simulink model "B_dot"  (Simulink 7.4)
settings: Solver=ode45  StartTime=0.0  StopTime=150000.0  RelTol=1e-3
libraries: aausat3_lib x8
settings Model: Creator=KFJensen  LastModifiedBy=kasperv
settings DataIOCC: LimitDataPoints=off
settings OptimizationCC: InlineParams=on  SimCompilerOptimization=On
settings DebuggingCC: SignalInfNanChecking=error  IntegerOverflowMsg=error  ParameterUnderflowMsg=error  AssertControl=DisableAll  StrictBusMsg=None
settings HardwareCC: ProdHWDeviceType=Generic->Unspecified (assume 32-bit Generic)

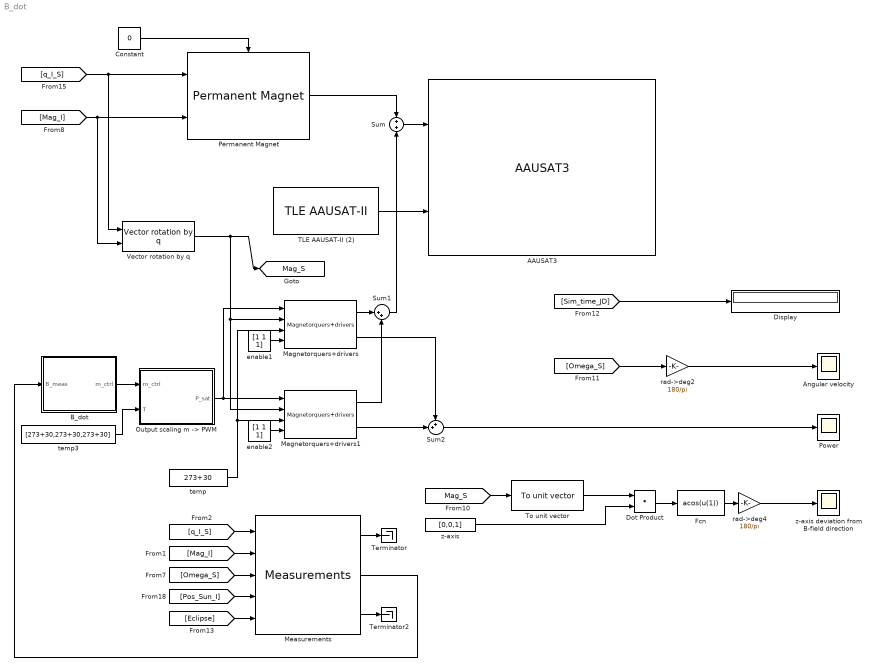
== system B_dot ==
  AAUSAT3 : aausat3_lib/AAUSAT3  SystemSampleTime=-1  r_com_s=[0.049073,0.048909,0.042976]  sat_temp_start=293.15  mass_sc=0.957820  Dim=[0.1,0.1,0.11]  inertia_c=[0.0017464,0.0022092,0.0022388]  init_jd=2455153.1954318  q_s_c=[-0.020656,0.71468,-0.007319,0.6991]  q_init_I_S=[1 0 0 0]  w_init_s=[1,1,1]*10*pi/180  Cd=2  rho=5e-14  solar_m_flux=4.5565e-6  solar_absorb_coeff=1.5  theta_e=65  refldata=load('lib/AlbedoToolbox-1.0/refl_data/2005/ga050101-051231')  redfac=1  Ts=1  enable_sensor_emulation=on  enable_env_disturbance=on
  Angular velocity : Scope
      settings: TimeRange=48000  YMin=-1  YMax=1  SaveName=ScopeData2  SampleInput=on
  B_dot : Subsystem  AncestorBlock=aausat3_lib/ACS/B_dot  mask{C=6000, wc=0.7, m_pm=-0.0030, Ts=0.1}
      mask prompts: C "Gain:"; wc "Filter cutoff frequency:"; m_pm "Permanent magnet dipole moment:"; Ts "Sample time:"
  Constant : Constant  Value=0  OutDataType=fixdt(1, 16)  OutScaling=2^0
  Display : Display
  Dot Product : DotProduct  OutDataType=fixdt(1, 16)  OutScaling=2^-10  InputSameDT=on  OutDataTypeStr=Inherit: Inherit via internal rule
  Fcn : Fcn  Expr=acos(u(1))
  Magnetorquers+drivers : aausat3_lib/Actuator Emulation/Magnetorquers+drivers  SystemSampleTime=-1  coil_dim=[0.075,0.075]  n_mt=250  A_wire_mt=(pi/4)*(0.13e-3)^2  sigma_0_mt=1.7e-8  alpha_0_mt=3.9e-3  T_0_mt=293.15  freq_mag=10  duty_mag=88
  Magnetorquers+drivers1 : aausat3_lib/Actuator Emulation/Magnetorquers+drivers  SystemSampleTime=-1  coil_dim=[0.075,0.075]  n_mt=250  A_wire_mt=(pi/4)*(0.13e-3)^2  sigma_0_mt=1.7e-8  alpha_0_mt=3.9e-3  T_0_mt=293.15  freq_mag=10  duty_mag=88
  Measurements : aausat3_lib/Sensor Emulation/Measurements  SystemSampleTime=-1  s_freq_mag=10  noise_mag=3  bias_mag=[0 0 0]  heading_mag=0  tilt_mag=0  s_freq_sun=1  noise_sun=3.33  bias_sun=[0 0]  nr_sample_sun=1  s_freq_gyro=1  noise_gyro=0.2  bias_gyro=[0 0 0]  heading_gyro=0  tilt_gyro=0
  "Output scaling m -> PWM" : Subsystem  AncestorBlock=aausat3_lib/Actuator Emulation/Output scaling m -> PWM  mask{coil_dim=[0.075,0.075], n_mt=250, A_wire_mt=(pi/4)*(0.13e-3)^2, sigma_0_mt=1.7e-8, alpha_0_mt=3.9e-3, T_0_mt=293.15, PWM_max=62.5, PWM_min=37.5}
      mask prompts: coil_dim "Coil Dimensions [x,y][m]:"; n_mt "Coil Winding Number [-]:"; A_wire_mt "Wire Cross Sectional Area [m^2]:"; sigma_0_mt "Wire Resistivity [Ohm*m]:"; alpha_0_mt "Wire Resistivity Temperature Coefficient [(deg C)^-1]:"; T_0_mt "Wire Resistivity Base Temperature [K]:"; PWM_max "PWM max [%]"; PWM_min "PWM min [%]"
  Permanent Magnet : aausat3_lib/Actuator Emulation/Permanent Magnet  SystemSampleTime=-1  mag_moment=-0.0030
  Power : Scope
      settings: TimeRange=48000  YMin=0  YMax=0.035  SaveName=ScopeData3  SampleInput=on
  Sum : Sum  OutDataType=fixdt(1, 16)  OutScaling=2^0
  Sum1 : Sum  Inputs=|++  OutDataType=fixdt(1, 16)  OutScaling=2^0
  Sum2 : Sum  Inputs=++|  OutDataType=fixdt(1, 16)  OutScaling=2^0
  TLE AAUSAT-II (2) : aausat3_lib/Orbit and Ephemeris/TLE AAUSAT-II  SystemSampleTime=-1  satname='AAUSAT-II'  JulianDay=09321.69542252  xndt2o=0.00000555  xndd6o=0.0  bstar=.76898e-4  xincl=97.9251  xnodeo=24.1597  eo=0.0014245  omegao=254.1774  xmo=105.7862  xno=14.81823818  ts=1
  Terminator : Terminator
  Terminator2 : Terminator
  To unit vector : aausat3_lib/Math Utilities/Vector operations/To unit vector  SystemSampleTime=-1
  Vector rotation by q : aausat3_lib/Actuator Emulation/Permanent Magnet/Vector rotation by q  SystemSampleTime=-1
  enable1 : Constant  Value=[1 1 1]  OutDataType=fixdt(1, 16)  OutScaling=2^0
  enable2 : Constant  Value=[1 1 1]  VectorParams1D=off  OutDataType=fixdt(1, 16)  OutScaling=2^0
  rad->deg2 : Gain  Gain=180/pi  ParameterDataType=fixdt(1, 16)  ParameterScaling=2^0  OutDataType=fixdt(1, 16)  OutScaling=2^0
  rad->deg4 : Gain  Gain=180/pi  ParameterDataType=fixdt(1, 16)  ParameterScaling=2^0  OutDataType=fixdt(1, 16)  OutScaling=2^0
  temp : Constant  Value=273+30  OutDataType=fixdt(1, 16)  OutScaling=2^0
  temp3 : Constant  Value=[273+30,273+30,273+30]  OutDataType=fixdt(1, 16)  OutScaling=2^0
  z-axis : Constant  Value=[0,0,1]  OutDataType=fixdt(1, 16)  OutScaling=2^0
  z-axis deviation from B-field direction : Scope
      settings: TimeRange=48000  YMin=0  YMax=180  SaveName=ScopeData9  SampleInput=on  SampleTime=1
  tag scope: Mag_S=global
  wires:
  TLE AAUSAT-II (2)/1 -> AAUSAT3/2
  [q_I_S] -> Permanent Magnet/1, Vector rotation by q/1
  [Mag_I] -> Permanent Magnet/2, Vector rotation by q/2
  Constant/1 -> Permanent Magnet/Enable
  [q_I_S] -> Measurements/1
  [Mag_I] -> Measurements/2
  [Omega_S] -> Measurements/3
  [Sim_time_JD] -> Display/1
  [Eclipse] -> Measurements/5
  [Pos_Sun_I] -> Measurements/4
  Sum/1 -> AAUSAT3/1
  Measurements/1 -> Terminator/1
  Measurements/3 -> Terminator2/1
  Permanent Magnet/1 -> Sum/1
  [Omega_S] -> rad->deg2/1
  rad->deg2/1 -> Angular velocity/1
  Sum1/1 -> Sum/2
  Vector rotation by q/1 -> [Mag_S], Magnetorquers+drivers/2, Magnetorquers+drivers1/2
  B_dot/1(m_ctrl) -> "Output scaling m -> PWM"/1(m_ctrl)
  "Output scaling m -> PWM"/1(P_sat) -> Magnetorquers+drivers/1, Magnetorquers+drivers1/1
  enable1/1 -> Magnetorquers+drivers/4
  enable2/1 -> Magnetorquers+drivers1/4
  temp/1 -> Magnetorquers+drivers/3, Magnetorquers+drivers1/3
  temp3/1 -> "Output scaling m -> PWM"/2(T)
  Magnetorquers+drivers/1 -> Sum1/1
  Magnetorquers+drivers1/1 -> Sum1/2
  Measurements/2 -> B_dot/1(B_meas)
  Magnetorquers+drivers1/2 -> Sum2/2
  Magnetorquers+drivers/2 -> Sum2/1
  Sum2/1 -> Power/1
  z-axis/1 -> Dot Product/2
  Dot Product/1 -> Fcn/1
  Fcn/1 -> rad->deg4/1
  rad->deg4/1 -> z-axis deviation from B-field direction/1
  To unit vector/1 -> Dot Product/1
  [Mag_S] -> To unit vector/1

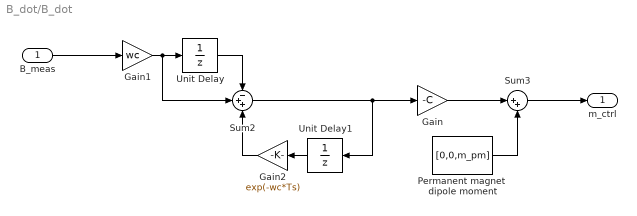
== system B_dot/B_dot ==
  B_meas : Inport  OutDataType=sfix(16)  OutScaling=2^0
  Gain : Gain  Gain=-C  ParameterDataType=fixdt(1, 16)  ParameterScaling=2^0  OutDataType=fixdt(1, 16)  OutScaling=2^0
  Gain1 : Gain  Gain=wc  ParameterDataType=fixdt(1, 16)  ParameterScaling=2^0  OutDataType=fixdt(1, 16)  OutScaling=2^0
  Gain2 : Gain  Gain=exp(-wc*Ts)  ParameterDataType=fixdt(1, 16)  ParameterScaling=2^0  OutDataType=fixdt(1, 16)  OutScaling=2^0
  Permanent magnet  dipole moment : Constant  Value=[0,0,m_pm]  OutDataType=fixdt(1, 16)  OutScaling=2^0
  Sum2 : Sum  Inputs=-++  OutDataType=fixdt(1, 16)  OutScaling=2^0
  Sum3 : Sum  Inputs=|++  OutDataType=fixdt(1, 16)  OutScaling=2^0
  Unit Delay : UnitDelay  SampleTime=-1
  Unit Delay1 : UnitDelay  SampleTime=-1
  m_ctrl : Outport  PortDimensions=3  OutDataType=sfix(16)  OutScaling=2^0
  wires:
  Sum3/1 -> m_ctrl/1
  Gain/1 -> Sum3/1
  Permanent magnet  dipole moment/1 -> Sum3/2
  Sum2/1 -> Unit Delay1/1, Gain/1
  Unit Delay1/1 -> Gain2/1
  Gain2/1 -> Sum2/3
  Gain1/1 -> Sum2/2, Unit Delay/1
  Unit Delay/1 -> Sum2/1
  B_meas/1 -> Gain1/1

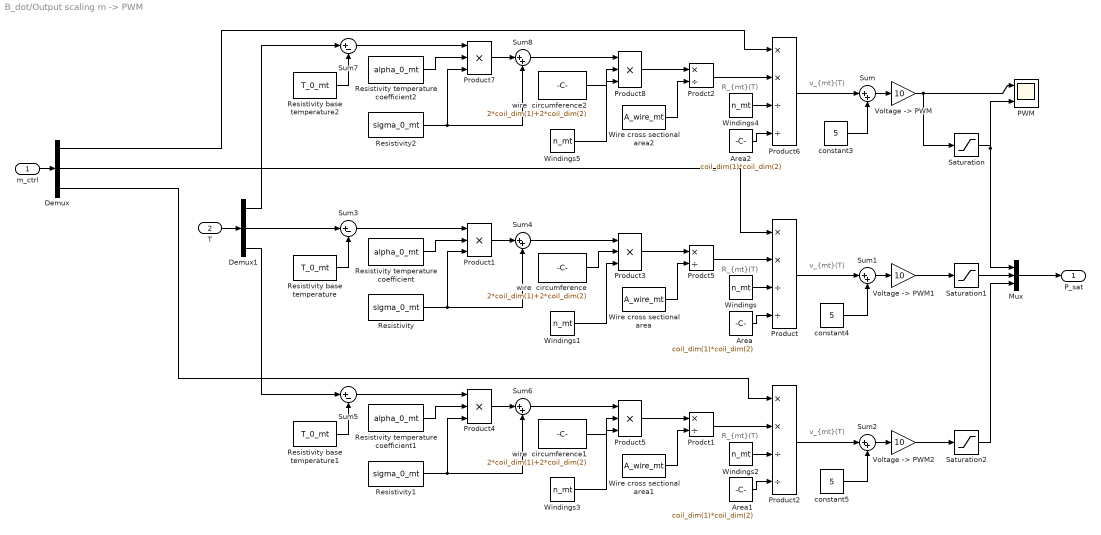
== system B_dot/Output scaling m -> PWM ==
  note: v_{mt}(T)
  note: v_{mt}(T)
  note: v_{mt}(T)
  note: R_{mt}(T)
  note: R_{mt}(T)
  note: R_{mt}(T)
  m_ctrl : Inport  OutDataType=sfix(16)  OutScaling=2^0
  T : Inport  Port=2  OutDataType=sfix(16)  OutScaling=2^0
  Area : Constant  Value=coil_dim(1)*coil_dim(2)  OutDataType=sfix(16)  OutScaling=2^0
  Area1 : Constant  Value=coil_dim(1)*coil_dim(2)  OutDataType=sfix(16)  OutScaling=2^0
  Area2 : Constant  Value=coil_dim(1)*coil_dim(2)  OutDataType=sfix(16)  OutScaling=2^0
  Demux : Demux  Outputs=3
  Demux1 : Demux  Outputs=3
  Mux : Mux  Inputs=3
  PWM : Scope  NumInputPorts=2
      settings: TimeRange=5000  YMin=37.5~37.5  YMax=67.5~62.5  SaveName=ScopeData4  SampleInput=on
  Prodct1 : Product  Inputs=*/  OutDataType=sfix(16)  OutScaling=2^0  RndMeth=Zero
  Prodct2 : Product  Inputs=*/  OutDataType=sfix(16)  OutScaling=2^0  RndMeth=Zero
  Prodct5 : Product  Inputs=*/  OutDataType=sfix(16)  OutScaling=2^0  RndMeth=Zero
  Product : Product  Inputs=**//  OutDataType=sfix(16)  OutScaling=2^0  RndMeth=Zero
  Product{1,3..5,7..8} (6 alike) : Product  Inputs=3  OutDataType=sfix(16)  OutScaling=2^0  RndMeth=Zero
  Product2 : Product  Inputs=**//  OutDataType=sfix(16)  OutScaling=2^0  RndMeth=Zero
  Product6 : Product  Inputs=**//  OutDataType=sfix(16)  OutScaling=2^0  RndMeth=Zero
  Resistivity : Constant  Value=sigma_0_mt  OutDataType=sfix(16)  OutScaling=2^0
  Resistivity base temperature : Constant  Value=T_0_mt  OutDataType=sfix(16)  OutScaling=2^0
  Resistivity base temperature1 : Constant  Value=T_0_mt  OutDataType=sfix(16)  OutScaling=2^0
  Resistivity base temperature2 : Constant  Value=T_0_mt  OutDataType=sfix(16)  OutScaling=2^0
  Resistivity temperature coefficient : Constant  Value=alpha_0_mt  OutDataType=sfix(16)  OutScaling=2^0
  Resistivity temperature coefficient1 : Constant  Value=alpha_0_mt  OutDataType=sfix(16)  OutScaling=2^0
  Resistivity temperature coefficient2 : Constant  Value=alpha_0_mt  OutDataType=sfix(16)  OutScaling=2^0
  Resistivity1 : Constant  Value=sigma_0_mt  OutDataType=sfix(16)  OutScaling=2^0
  Resistivity2 : Constant  Value=sigma_0_mt  OutDataType=sfix(16)  OutScaling=2^0
  Saturation : Saturate  UpperLimit=PWM_max  LowerLimit=PWM_min
  Saturation1 : Saturate  UpperLimit=PWM_max  LowerLimit=PWM_min
  Saturation2 : Saturate  UpperLimit=PWM_max  LowerLimit=PWM_min
  Sum : Sum  Inputs=|++  OutDataType=fixdt(1, 16)  OutScaling=2^0
  Sum1 : Sum  Inputs=|++  OutDataType=fixdt(1, 16)  OutScaling=2^0
  Sum2 : Sum  Inputs=|++  OutDataType=fixdt(1, 16)  OutScaling=2^0
  Sum3 : Sum  Inputs=|+-  OutDataType=sfix(16)  OutScaling=2^0
  Sum4 : Sum  Inputs=|++  OutDataType=sfix(16)  OutScaling=2^0
  Sum5 : Sum  Inputs=|+-  OutDataType=sfix(16)  OutScaling=2^0
  Sum6 : Sum  Inputs=|++  OutDataType=sfix(16)  OutScaling=2^0
  Sum7 : Sum  Inputs=|+-  OutDataType=sfix(16)  OutScaling=2^0
  Sum8 : Sum  Inputs=|++  OutDataType=sfix(16)  OutScaling=2^0
  "Voltage -> PWM" : Gain  Gain=10  ParameterDataType=fixdt(1, 16)  ParameterScaling=2^0  OutDataType=fixdt(1, 16)  OutScaling=2^0
  "Voltage -> PWM1" : Gain  Gain=10  ParameterDataType=fixdt(1, 16)  ParameterScaling=2^0  OutDataType=fixdt(1, 16)  OutScaling=2^0
  "Voltage -> PWM2" : Gain  Gain=10  ParameterDataType=fixdt(1, 16)  ParameterScaling=2^0  OutDataType=fixdt(1, 16)  OutScaling=2^0
  Windings{,1..5} (6 alike) : Constant  Value=n_mt  OutDataType=sfix(16)  OutScaling=2^0
  Wire cross sectional area : Constant  Value=A_wire_mt  OutDataType=sfix(16)  OutScaling=2^0
  Wire cross sectional area1 : Constant  Value=A_wire_mt  OutDataType=sfix(16)  OutScaling=2^0
  Wire cross sectional area2 : Constant  Value=A_wire_mt  OutDataType=sfix(16)  OutScaling=2^0
  constant3 : Constant  Value=5  OutDataType=sfix(16)  OutScaling=2^0
  constant4 : Constant  Value=5  OutDataType=sfix(16)  OutScaling=2^0
  constant5 : Constant  Value=5  OutDataType=sfix(16)  OutScaling=2^0
  wire  circumference : Constant  Value=2*coil_dim(1)+2*coil_dim(2)  OutDataType=sfix(16)  OutScaling=2^0
  wire  circumference1 : Constant  Value=2*coil_dim(1)+2*coil_dim(2)  OutDataType=sfix(16)  OutScaling=2^0
  wire  circumference2 : Constant  Value=2*coil_dim(1)+2*coil_dim(2)  OutDataType=sfix(16)  OutScaling=2^0
  P_sat : Outport  PortDimensions=3  OutDataType=sfix(16)  OutScaling=2^0
  wires:
  Product2/1 -> Sum2/1
  Product/1 -> Sum1/1
  Product6/1 -> Sum/1
  Demux/3 -> Product2/1
  Demux/2 -> Product/1
  Demux/1 -> Product6/1
  "Voltage -> PWM2"/1 -> Saturation2/1
  "Voltage -> PWM1"/1 -> Saturation1/1
  "Voltage -> PWM"/1 -> Saturation/1, PWM/1
  Area2/1 -> Product6/4
  Windings4/1 -> Product6/3
  Area1/1 -> Product2/4
  Windings2/1 -> Product2/3
  Area/1 -> Product/4
  Windings/1 -> Product/3
  T/1 -> Demux1/1
  Sum2/1 -> "Voltage -> PWM2"/1
  Sum1/1 -> "Voltage -> PWM1"/1
  Sum/1 -> "Voltage -> PWM"/1
  Saturation2/1 -> Mux/3
  Saturation1/1 -> Mux/2
  Saturation/1 -> Mux/1, PWM/2
  Mux/1 -> P_sat/1
  m_ctrl/1 -> Demux/1
  constant3/1 -> Sum/2
  constant4/1 -> Sum1/2
  constant5/1 -> Sum2/2
  Wire cross sectional area1/1 -> Prodct1/2
  Product5/1 -> Prodct1/1
  Windings3/1 -> Product5/3
  wire  circumference1/1 -> Product5/2
  Sum6/1 -> Product5/1
  Product4/1 -> Sum6/1
  Resistivity1/1 -> Sum6/2, Product4/3
  Sum5/1 -> Product4/1
  Resistivity temperature coefficient1/1 -> Product4/2
  Resistivity base temperature1/1 -> Sum5/2
  Demux1/3 -> Sum5/1
  Demux1/2 -> Sum3/1
  Wire cross sectional area/1 -> Prodct5/2
  Product3/1 -> Prodct5/1
  Windings1/1 -> Product3/3
  wire  circumference/1 -> Product3/2
  Sum4/1 -> Product3/1
  Product1/1 -> Sum4/1
  Resistivity/1 -> Sum4/2, Product1/3
  Sum3/1 -> Product1/1
  Resistivity temperature coefficient/1 -> Product1/2
  Resistivity base temperature/1 -> Sum3/2
  Demux1/1 -> Sum7/1
  Wire cross sectional area2/1 -> Prodct2/2
  Product8/1 -> Prodct2/1
  Windings5/1 -> Product8/3
  wire  circumference2/1 -> Product8/2
  Sum8/1 -> Product8/1
  Product7/1 -> Sum8/1
  Resistivity2/1 -> Sum8/2, Product7/3
  Sum7/1 -> Product7/1
  Resistivity temperature coefficient2/1 -> Product7/2
  Resistivity base temperature2/1 -> Sum7/2
  Prodct1/1 -> Product2/2
  Prodct5/1 -> Product/2
  Prodct2/1 -> Product6/2
